simulink model "GradientIdentifier_DREM"  (R2021a)
settings: Solver=VariableStepAuto  StartTime=0.0  StopTime=20  RelTol=1e-3
libraries: simulink x4
settings Model: Creator=simon  LastModifiedBy=simon
settings SolverCC: AlgebraicLoopSolver=TrustRegion

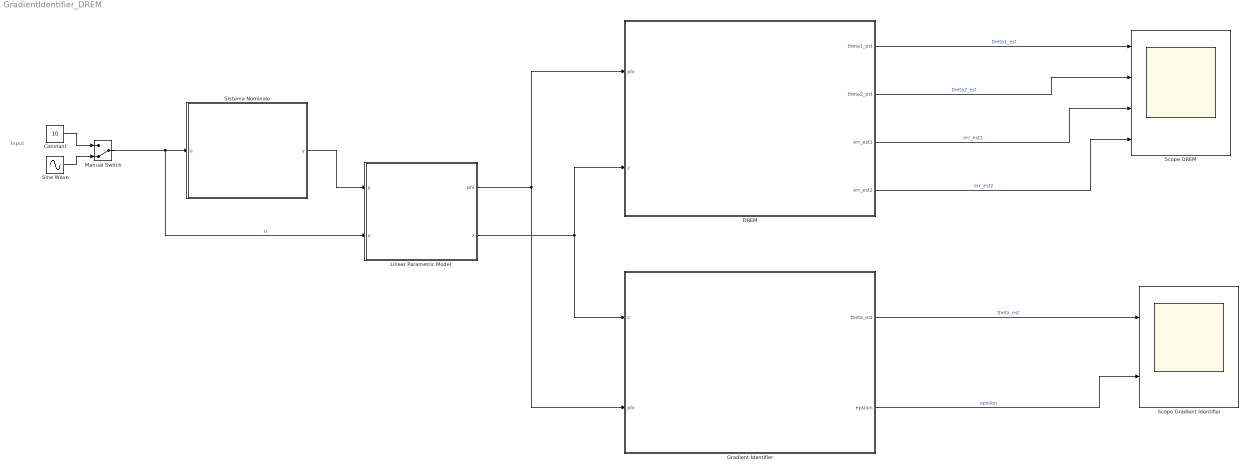
== system GradientIdentifier_DREM ==
  note: Input
  Constant : Constant  Value=10
  "DREM " : Subsystem
  Gradient Identifier : Subsystem
  Linear Parametric Model : Subsystem
  Manual Switch : ManualSwitch  CurrentSetting=0
  Scope DREM : Scope  NumInputPorts=4
  Scope Gradient Identifier : Scope  NumInputPorts=2
  Sine Wave : Sin  Amplitude=10  Frequency=5/2  SampleTime=0
  Sistema Nominale : Subsystem
  wires:
  Sine Wave/1 -> Manual Switch/2
  Constant/1 -> Manual Switch/1
  Manual Switch/1 -> Linear Parametric Model/2(u), Sistema Nominale/1(u)  "u"
  Sistema Nominale/1(y) -> Linear Parametric Model/1(y)
  Linear Parametric Model/2(z) -> Gradient Identifier/1(z), "DREM "/2(z)
  Linear Parametric Model/1(phi) -> Gradient Identifier/2(phi), "DREM "/1(phi)
  "DREM "/1(theta1_est) -> Scope DREM/1  "theta1_est"
  "DREM "/2(theta2_est) -> Scope DREM/2  "theta2_est"
  "DREM "/3(err_est1) -> Scope DREM/3  "err_est1"
  "DREM "/4(err_est2) -> Scope DREM/4  "err_est2"
  Gradient Identifier/1(theta_est) -> Scope Gradient Identifier/1  "theta_est"
  Gradient Identifier/2(epsilon) -> Scope Gradient Identifier/2  "epsilon"

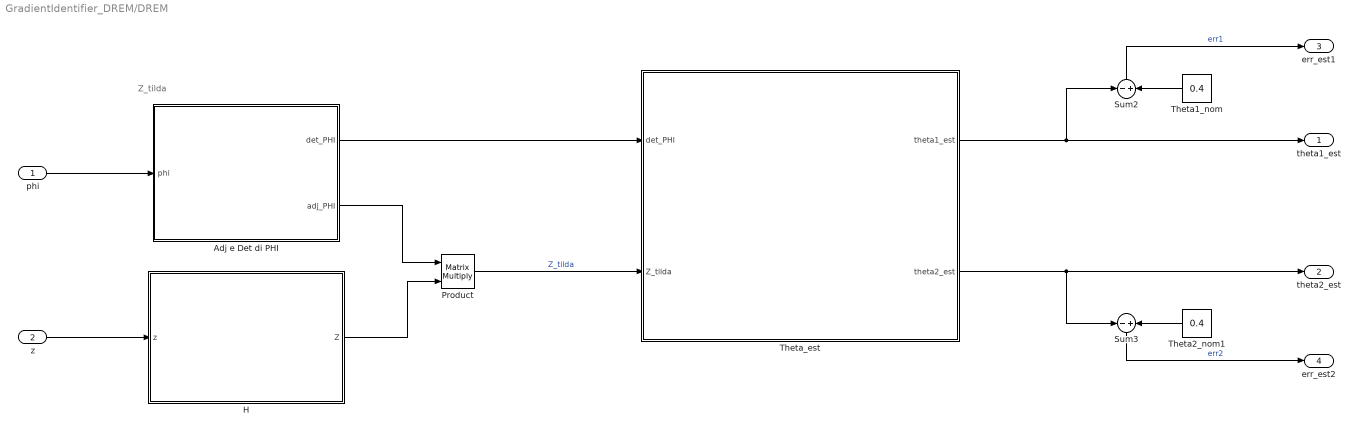
== system GradientIdentifier_DREM/DREM  ==
  note: Z_tilda
  phi : Inport
  z : Inport  Port=2
  Adj e Det di PHI : Subsystem
  H : Subsystem
  Product : Product  Multiplication=Matrix(*)
  Sum2 : Sum  Inputs=-+
  Sum3 : Sum  Inputs=-+
  Theta1_nom : Constant  Value=0.4
  Theta2_nom1 : Constant  Value=0.4
  Theta_est : Subsystem
  theta1_est : Outport
  theta2_est : Outport  Port=2
  err_est1 : Outport  Port=3
  err_est2 : Outport  Port=4
  wires:
  Theta1_nom/1 -> Sum2/2
  Theta2_nom1/1 -> Sum3/2
  z/1 -> H/1(z)
  H/1(Z) -> Product/2
  Adj e Det di PHI/2(adj_PHI) -> Product/1
  phi/1 -> Adj e Det di PHI/1(phi)
  Theta_est/2(theta2_est) -> theta2_est/1, Sum3/1
  Theta_est/1(theta1_est) -> theta1_est/1, Sum2/1
  Adj e Det di PHI/1(det_PHI) -> Theta_est/1(det_PHI)
  Product/1 -> Theta_est/2(Z_tilda)  "Z_tilda"
  Sum3/1 -> err_est2/1  "err2"
  Sum2/1 -> err_est1/1  "err1"

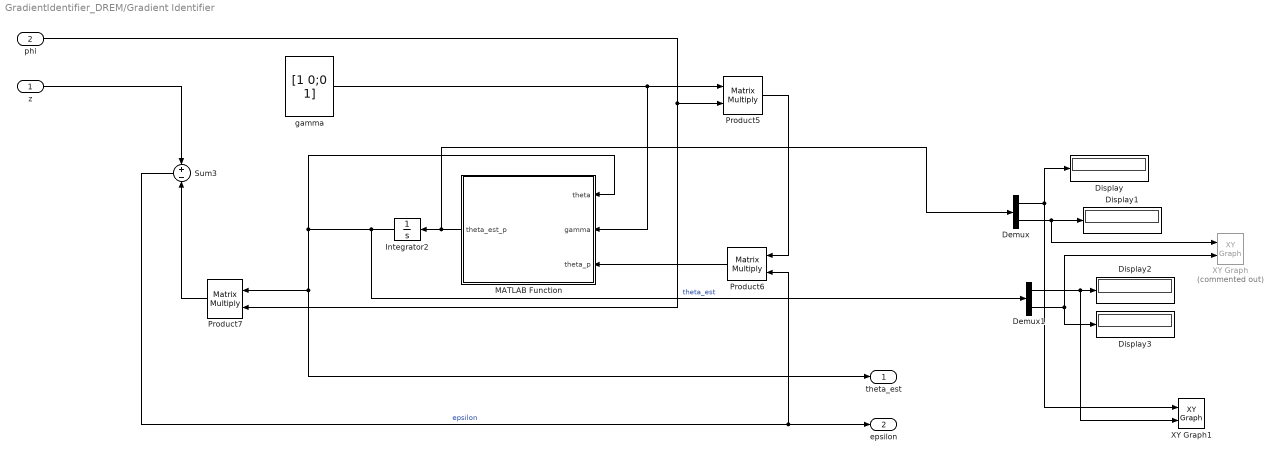
== system GradientIdentifier_DREM/Gradient Identifier ==
  z : Inport
  phi : Inport  Port=2
  Demux : Demux  Outputs=2
  Demux1 : Demux  Outputs=2
  Display{,1..3} (4 alike) : Display
  Integrator2 : Integrator  InitialCondition=1
  MATLAB Function : MATLAB Function  TreatAsAtomicUnit=on
  Product5 : Product  Multiplication=Matrix(*)
  Product6 : Product  Multiplication=Matrix(*)
  Product7 : Product  Multiplication=Matrix(*)
  Sum3 : Sum  Inputs=+-
  XY Graph : simulink/Sinks/XY Graph  Commented=on  xmin=-2  xmax=2  ymin=-2  ymax=2  st=-1
  XY Graph1 : simulink/Sinks/XY Graph  xmin=-2  xmax=2  ymin=-2  ymax=2  st=-1
  gamma : Constant  Value=[1 0;0 1]
  theta_est : Outport
  epsilon : Outport  Port=2
  wires:
  gamma/1 -> Product5/1, MATLAB Function/2(gamma)
  phi/1 -> Product7/2, Product5/2
  Product6/1 -> MATLAB Function/3(theta_p)
  Sum3/1 -> Product6/2, epsilon/1  "epsilon"
  Product5/1 -> Product6/1
  Integrator2/1 -> Demux1/1, MATLAB Function/1(theta), Product7/1, theta_est/1  "theta_est"
  MATLAB Function/1(theta_est_p) -> Demux/1, Integrator2/1
  Product7/1 -> Sum3/2
  z/1 -> Sum3/1
  Demux/2 -> XY Graph/1, Display1/1
  Demux/1 -> XY Graph1/1, Display/1
  Demux1/1 -> XY Graph1/2, Display2/1
  Demux1/2 -> XY Graph/2, Display3/1

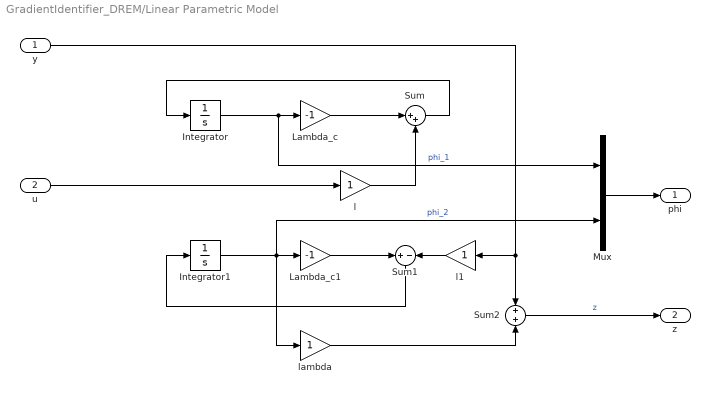
== system GradientIdentifier_DREM/Linear Parametric Model ==
  y : Inport
  u : Inport  Port=2
  Integrator : Integrator
  Integrator1 : Integrator
  Lambda_c : Gain  Gain=-1
  Lambda_c1 : Gain  Gain=-1
  Mux : Mux  Inputs=2
  Sum : Sum  Inputs=|++
  Sum1 : Sum  Inputs=+-
  Sum2 : Sum
  l : Gain
  l1 : Gain
  lambda : Gain
  phi : Outport
  z : Outport  Port=2
  wires:
  Sum1/1 -> Integrator1/1
  Integrator/1 -> Mux/1, Lambda_c/1  "phi_1"
  Integrator1/1 -> Mux/2, Lambda_c1/1, lambda/1  "phi_2"
  Sum/1 -> Integrator/1
  Lambda_c/1 -> Sum/1
  l/1 -> Sum/2
  Lambda_c1/1 -> Sum1/1
  lambda/1 -> Sum2/2
  l1/1 -> Sum1/2
  y/1 -> l1/1, Sum2/1
  Sum2/1 -> z/1  "z"
  u/1 -> l/1
  Mux/1 -> phi/1

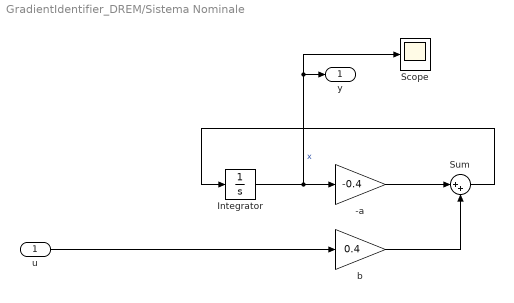
== system GradientIdentifier_DREM/Sistema Nominale ==
  u : Inport
  -a : Gain  Gain=-0.4
  Integrator : Integrator
  Scope : Scope
  Sum : Sum  Inputs=|++
  b : Gain  Gain=0.4
  y : Outport
  wires:
  -a/1 -> Sum/1
  b/1 -> Sum/2
  Integrator/1 -> Scope/1, y/1, -a/1  "x"
  Sum/1 -> Integrator/1
  u/1 -> b/1

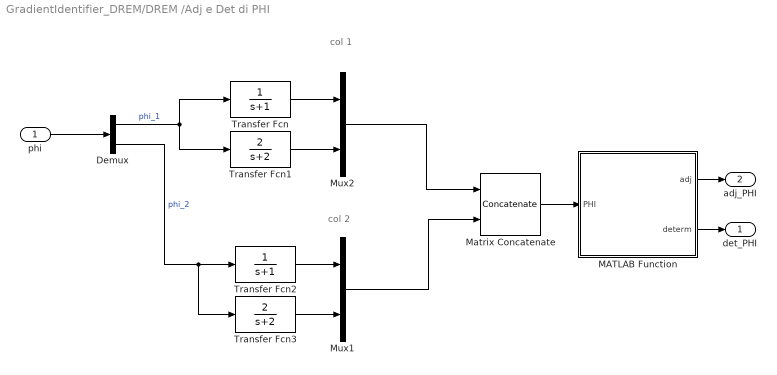
== system GradientIdentifier_DREM/DREM /Adj e Det di PHI ==
  note: col 2
  note: col 1
  phi : Inport
  Demux : Demux  Outputs=2
  MATLAB Function : MATLAB Function  TreatAsAtomicUnit=on
  Matrix Concatenate : Concatenate  Mode=Multidimensional array  ConcatenateDimension=2
  Mux1 : Mux  Inputs=2
  Mux2 : Mux  Inputs=2
  Transfer Fcn : TransferFcn  Denominator=[1 1]
  Transfer Fcn1 : TransferFcn  Numerator=[2]  Denominator=[1 2]
  Transfer Fcn2 : TransferFcn  Denominator=[1 1]
  Transfer Fcn3 : TransferFcn  Numerator=[2]  Denominator=[1 2]
  det_PHI : Outport
  adj_PHI : Outport  Port=2
  wires:
  Demux/1 -> Transfer Fcn1/1, Transfer Fcn/1  "phi_1"
  Demux/2 -> Transfer Fcn3/1, Transfer Fcn2/1  "phi_2"
  phi/1 -> Demux/1
  Transfer Fcn/1 -> Mux2/1
  Transfer Fcn2/1 -> Mux1/1
  Transfer Fcn3/1 -> Mux1/2
  Mux2/1 -> Matrix Concatenate/1
  Mux1/1 -> Matrix Concatenate/2
  Matrix Concatenate/1 -> MATLAB Function/1(PHI)
  MATLAB Function/1(adj) -> adj_PHI/1
  MATLAB Function/2(determ) -> det_PHI/1
  Transfer Fcn1/1 -> Mux2/2

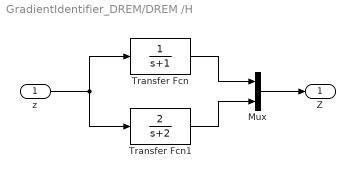
== system GradientIdentifier_DREM/DREM /H ==
  z : Inport
  Mux : Mux  Inputs=2
  Transfer Fcn : TransferFcn  Denominator=[1 1]
  Transfer Fcn1 : TransferFcn  Numerator=[2]  Denominator=[1 2]
  Z : Outport
  wires:
  z/1 -> Transfer Fcn1/1, Transfer Fcn/1
  Transfer Fcn/1 -> Mux/1
  Transfer Fcn1/1 -> Mux/2
  Mux/1 -> Z/1

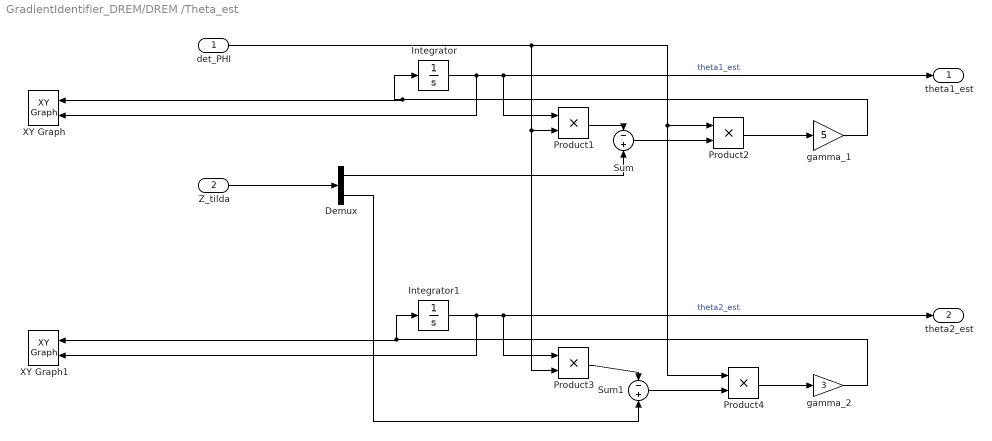
== system GradientIdentifier_DREM/DREM /Theta_est ==
  det_PHI : Inport
  Z_tilda : Inport  Port=2
  Demux : Demux  Outputs=2
  Integrator : Integrator
  Integrator1 : Integrator
  Product{1..4} (4 alike) : Product
  Sum : Sum  Inputs=-+
  Sum1 : Sum  Inputs=-+
  XY Graph : simulink/Sinks/XY Graph  xmin=-1  xmax=1  ymin=-1  ymax=1  st=-1
  XY Graph1 : simulink/Sinks/XY Graph  xmin=-1  xmax=1  ymin=-1  ymax=1  st=-1
  gamma_1 : Gain  Gain=5
  gamma_2 : Gain  Gain=3
  theta1_est : Outport
  theta2_est : Outport  Port=2
  wires:
  Product2/1 -> gamma_1/1
  Integrator1/1 -> XY Graph1/2, theta2_est/1, Product3/1  "theta2_est"
  Product1/1 -> Sum/1
  Demux/1 -> Sum/2
  gamma_1/1 -> XY Graph/1, Integrator/1
  det_PHI/1 -> Product3/2, Product1/2, Product4/1, Product2/1
  Integrator/1 -> XY Graph/2, theta1_est/1, Product1/1  "theta1_est"
  Demux/2 -> Sum1/2
  Product4/1 -> gamma_2/1
  Product3/1 -> Sum1/1
  Sum/1 -> Product2/2
  Sum1/1 -> Product4/2
  gamma_2/1 -> XY Graph1/1, Integrator1/1
  Z_tilda/1 -> Demux/1

== matlab function GradientIdentifier_DREM/Gradient Identifier/MATLAB Function ==
  data: theta input; gamma input; theta_est_p output; theta_p input
function theta_est_p = projection(theta,gamma,theta_p)

grad_G = [-1 0]';
eps = 1e-3;

g = -theta(1)+eps;
v = theta_p'*grad_G; % è scalare

if((g < 0) || ( g == 0 && v(1)<=0))
    theta_est_p =  theta_p;
else
    theta_est_p = theta_p - gamma*grad_G*inv(grad_G'*gamma*grad_G)*grad_G'*theta_p;
end

end

== matlab function GradientIdentifier_DREM/DREM /Adj e Det di PHI/MATLAB Function ==
  data: PHI input; adj output; determ output
function [adj,determ] = adjoint(PHI)
determ = det(PHI);
adj = [PHI(2,2) -PHI(1,2);-PHI(2,1) PHI(1,1)];
end
